simulink model "ADC_example1"  (Simulink 7.7)
settings: Solver=ode45  StartTime=0.0  StopTime=T  MaxStep=MaxStep  RelTol=RelTol
values from neighbouring files (symbols this model uses):
  J = 20    [initialization_exADC.m]
  rule = 1    [initialization_exADC.m]
  T = 10    [initialization_exADC.m]
  x0ADC = [0;0]    [initialization_exADC.m]
libraries: simulink x3
settings Model: Creator=pablonanez  LastModifiedBy=pablonanez

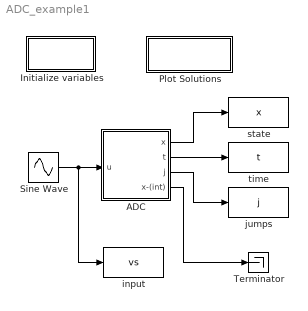
== system ADC_example1 ==
  ADC : Subsystem  LoadFcn=set_param(gcb,'LinkStatus','none')
      settings: CopyFcn=|
      | set_param(gcb,'LinkStatus','none'),
      | set_param(gcs, 'MaxStep', 'MaxStep', 'RelTol', 'RelTol','Stop time', 'T')
      mask Display:
      | image(imread('ADC.jpg'))
      | %plot([5 20 20 5 5],[5 5 20 20 5])
      | %text(8,13,'HyEq_mdl')
      | port_label('output', 1, 'x')
      | port_label('output', 2, 't')
      | port_label('output', 3, 'j')
      | port_label('output', 4, 'x-(int)')
      | port_label('input', 1, 'u')
  Initialize variables : Subsystem  Priority=-10
      settings: OpenFcn=initialization_exADC
      mask Display: disp('Double Click\n to Initialize')
  Plot Solutions : Subsystem
      settings: OpenFcn=postprocessing_exADC
      mask Display: disp('Double Click to\n Plot Solutions')
  Sine Wave : Sin  SampleTime=0
  Terminator : Terminator
  input : ToWorkspace  VariableName=vs  SampleTime=-1  SaveFormat=Array
  jumps : ToWorkspace  VariableName=j  SampleTime=-1  SaveFormat=Array
  state : ToWorkspace  VariableName=x  SampleTime=-1  SaveFormat=Array
  time : ToWorkspace  VariableName=t  SampleTime=-1  SaveFormat=Array
  wires:
  Sine Wave/1 -> ADC/1(u), input/1
  ADC/1(x) -> state/1
  ADC/2(t) -> time/1
  ADC/3(j) -> jumps/1
  ADC/4(x-(int)) -> Terminator/1

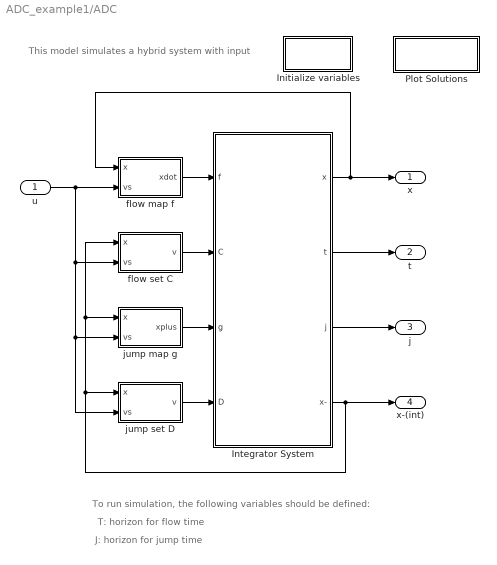
== system ADC_example1/ADC ==
  note: J: horizon for jump time
  note: T: horizon for flow time
  note: To run simulation, the following variables should be defined:
  note: This model simulates a hybrid system with input
  u : Inport
  Initialize variables : Subsystem  Priority=-10
      settings: OpenFcn=|
      | try
      |      clearvars -except inifile pathfile_in pathfile_pos posfile
      |      cd(pathfile_in);
      |      eval(inifile);
      | catch
      |      [inifile,pathfile_in] = getInitializationfile;
      |      cd(pathfile_in);
      |      inifile = strrep(inifile,'.m','');
      |      eval(inifile);
      | end
      mask Display: disp('Double Click\n to Initialize')
  Integrator System : Subsystem  Priority=2  mask(Hybrid Integrator){T=T, J=J, x0=x0ADC}
      mask prompts: T "Flow Horizon"; J "Jump Horizon"; x0 "Initial Condition"
      mask help:
      | This block integrates the state of the hybrid system defined by the flow map f (first input), the flow set C (second input), the jump map g (third input) and the jump set D (fourth input).
      | Starting from the initial condition x0 (last mask parameter), the system's state x evolves continuously within the set C, according to f(x,u), but is also subject to jumps within D, according to g(x,u).
      | The block also stops the simulation when the time t is greater than the flow horizon T (first mask parameter), or when the number of jumps j is greater than the jump horizon J (second mask parameter).
      | The outputs of the blocks are respectively x(t), t, j, x(t-).
      mask Help:
      | This block integrates the state of the hybrid system defined by the flow map f (first input), the flow set C (second input), the jump map g (third input) and the jump set D (fourth input).
      | <br>
      | Starting from the initial condition x0 (last mask parameter), the system's state x evolves continuously within the set C, according to f(x,u), but is also subject to jumps within D, according to g(x,u).
      | <br>
      | The block also stops the simulation when the time t is greater than the flow horizon T (first mask parameter), or when the number of jumps j is greater than the jump horizon J (second mask parameter).
      | <br>
      | The outputs of the blocks are respectively x(t), t, j, x(t-).
      | <br>
      | You can right click on the block and "Look under mask" to see what's inside the block.
      | Finally, refer to the manual (HybridSimulator_vXX.pdf) for more detailed information on how this hybrid simulator works.
  Plot Solutions : Subsystem
      settings: OpenFcn=|
      | try
      |      cd(pathfile_pos);
      |      eval(posfile);
      | catch
      |      [posfile,pathfile_pos] = getInitializationfile;
      |      cd(pathfile_pos);
      |      posfile = strrep(posfile,'.m','');
      |      eval(posfile);
      | end
      mask Display: disp('Double Click to\n Plot Solutions')
  flow map f : Stateflow chart  TreatAsAtomicUnit=on
  flow set C : Stateflow chart  TreatAsAtomicUnit=on
  jump map g : Stateflow chart  Priority=2  TreatAsAtomicUnit=on
  jump set D : Stateflow chart  TreatAsAtomicUnit=on
  x : Outport
  t : Outport  Port=2
  j : Outport  Port=3
  x-(int) : Outport  Port=4
  wires:
  jump map g/1(xplus) -> Integrator System/3(g)
  jump set D/1(v) -> Integrator System/4(D)
  u/1 -> jump set D/2(vs), jump map g/2(vs), flow set C/2(vs), flow map f/2(vs)
  Integrator System/3(j) -> j/1
  Integrator System/2(t) -> t/1
  flow set C/1(v) -> Integrator System/2(C)
  Integrator System/1(x) -> x/1, flow map f/1(x)
  Integrator System/4(x-) -> x-(int)/1, jump set D/1(x), flow set C/1(x), jump map g/1(x)
  flow map f/1(xdot) -> Integrator System/1(f)

== system ADC_example1/Initialize variables ==

== system ADC_example1/Plot Solutions ==

== system ADC_example1/ADC/Initialize variables ==

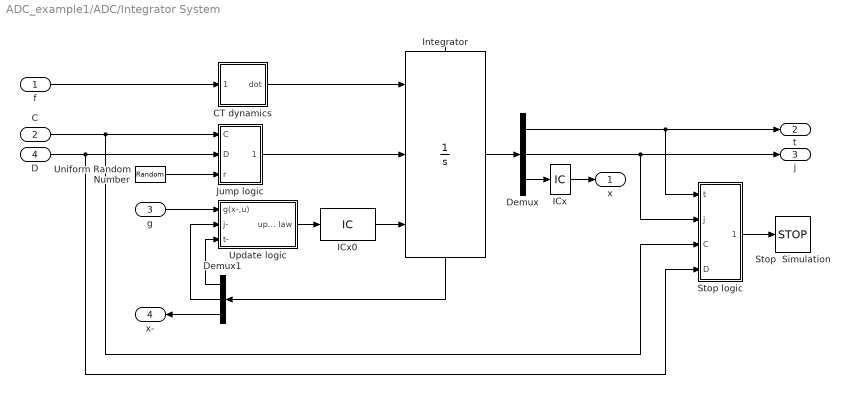
== system ADC_example1/ADC/Integrator System ==
  f : Inport
  C : Inport  Port=2
  g : Inport  Port=3
  D : Inport  Port=4
  CT dynamics : Subsystem
  Demux : Demux  Outputs=[1 1 -1]
  Demux1 : Demux  Outputs=[1 1 -1]
  ICx : InitialCondition  Value=x0
  ICx0 : InitialCondition  Value=[0; 0; x0(:)]
  Integrator : Integrator  ExternalReset=level hold  InitialConditionSource=external  ShowStatePort=on  ZeroCross=off
  Jump logic : Subsystem
  Stop  Simulation : Stop
  Stop logic : Subsystem
  Uniform Random Number : UniformRandomNumber  Minimum=0  Seed=abs(floor(100*rand))  SampleTime=0
  Update logic : Subsystem
  x : Outport
  t : Outport  Port=2
  j : Outport  Port=3
  x- : Outport  Port=4
  wires:
  ICx0/1 -> Integrator/3
  ICx/1 -> x/1
  Demux/3 -> ICx/1
  Integrator/State -> Demux1/1
  Demux/2 -> j/1, Stop logic/2(j)
  Demux/1 -> t/1, Stop logic/1(t)
  Update logic/1(update law) -> ICx0/1
  CT dynamics/1(dot) -> Integrator/1
  Stop logic/1(stop) -> Stop  Simulation/1
  Integrator/1 -> Demux/1
  C/1 -> Stop logic/3(C), Jump logic/1(C)
  D/1 -> Stop logic/4(D), Jump logic/2(D)
  f/1 -> CT dynamics/1(f(x,u))
  Demux1/3 -> x-/1
  Jump logic/1(jump) -> Integrator/2
  Uniform Random Number/1 -> Jump logic/3(r)
  g/1 -> Update logic/1(g(x-,u))
  Demux1/1 -> Update logic/3(t-)
  Demux1/2 -> Update logic/2(j-)

== system ADC_example1/ADC/Plot Solutions ==

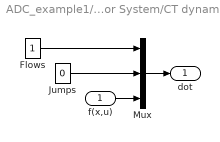
== system ADC_example1/ADC/Integrator System/CT dynamics ==
  f(x,u) : Inport
  Flows : Constant
  Jumps : Constant  Value=0
  Mux : Mux  Inputs=[1 1 -1]
  dot : Outport
  wires:
  Jumps/1 -> Mux/2
  Flows/1 -> Mux/1
  Mux/1 -> dot/1
  f(x,u)/1 -> Mux/3

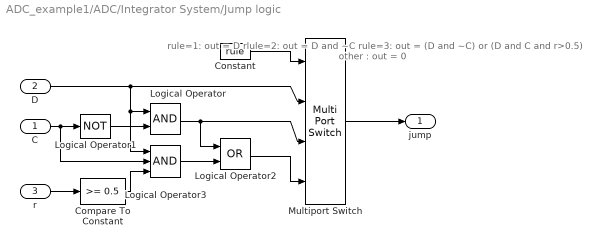
== system ADC_example1/ADC/Integrator System/Jump logic ==
  note: rule=1:  out = D
      | rlule=2: out = D and ~C
      | rule=3:  out = (D and ~C)  or (D and C and r>0.5)
      | other :  out = 0
  C : Inport
  D : Inport  Port=2
  r : Inport  Port=3
  Compare To Constant : simulink/Logic and Bit Operations/Compare To Constant  SystemSampleTime=-1  relop=>=  const=0.5  LogicOutDataTypeMode=uint8
  Constant : Constant  Value=rule
  Logical Operator : Logic  AllPortsSameDT=off  OutDataTypeStr=boolean
  Logical Operator1 : Logic  Operator=NOT  Inputs=1  AllPortsSameDT=off  OutDataTypeStr=boolean
  Logical Operator2 : Logic  Operator=OR  AllPortsSameDT=off  OutDataTypeStr=boolean
  Logical Operator3 : Logic  Inputs=3  AllPortsSameDT=off  OutDataTypeStr=boolean
  Multiport Switch : MultiPortSwitch  zeroidx=off
  jump : Outport
  wires:
  Constant/1 -> Multiport Switch/1
  D/1 -> Logical Operator3/1, Logical Operator/1, Multiport Switch/2
  r/1 -> Compare To Constant/1
  C/1 -> Logical Operator3/2, Logical Operator1/1
  Logical Operator1/1 -> Logical Operator/2
  Logical Operator/1 -> Multiport Switch/3, Logical Operator2/1
  Logical Operator2/1 -> Multiport Switch/4
  Multiport Switch/1 -> jump/1
  Compare To Constant/1 -> Logical Operator3/3
  Logical Operator3/1 -> Logical Operator2/2

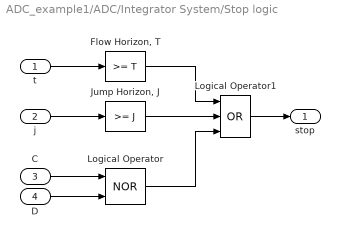
== system ADC_example1/ADC/Integrator System/Stop logic ==
  t : Inport
  j : Inport  Port=2
  C : Inport  Port=3
  D : Inport  Port=4
  "Flow Horizon, T" : simulink/Logic and Bit Operations/Compare To Constant  SystemSampleTime=-1  relop=>=  const=T  LogicOutDataTypeMode=uint8  ZeroCross=off
  "Jump Horizon, J" : simulink/Logic and Bit Operations/Compare To Constant  SystemSampleTime=-1  relop=>=  const=J  LogicOutDataTypeMode=uint8  ZeroCross=off
  Logical Operator : Logic  Operator=NOR  AllPortsSameDT=off  OutDataTypeStr=boolean
  Logical Operator1 : Logic  Operator=OR  Inputs=3  AllPortsSameDT=off  OutDataTypeStr=boolean
  stop : Outport
  wires:
  "Flow Horizon, T"/1 -> Logical Operator1/1
  "Jump Horizon, J"/1 -> Logical Operator1/2
  Logical Operator/1 -> Logical Operator1/3
  D/1 -> Logical Operator/2
  t/1 -> "Flow Horizon, T"/1
  j/1 -> "Jump Horizon, J"/1
  C/1 -> Logical Operator/1
  Logical Operator1/1 -> stop/1

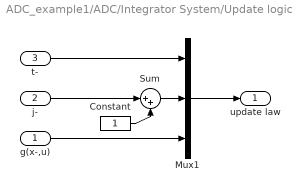
== system ADC_example1/ADC/Integrator System/Update logic ==
  g(x-,u) : Inport
  j- : Inport  Port=2
  t- : Inport  Port=3
  Constant : Constant
  Mux1 : Mux  Inputs=[1 1 -1]
  Sum : Sum  Inputs=|++
  update law : Outport
  wires:
  Sum/1 -> Mux1/2
  Mux1/1 -> update law/1
  j-/1 -> Sum/1
  g(x-,u)/1 -> Mux1/3
  t-/1 -> Mux1/1
  Constant/1 -> Sum/2

== matlab function ADC/flow map f ==
  data: x input double; xdot output double; vs input double
function xdot = f(x,vs)
%--------------------------------------------------------------------------
% Matlab M-file Project: HyEQ Toolbox @  Hybrid Systems Laboratory (HSL), 
% https://hybrid.soe.ucsc.edu/software
% http://hybridsimulator.wordpress.com/
%--------------------------------------------------------------------------
% Project: Simulation of a hybrid system Analog-to-Digital converter (ADC) 
% Description: Flow map
%--------------------------------------------------------------------------
%--------------------------------------------------------------------------
%   See also plotflows, plotHarc, plotHarcColor, plotHarcColor3D,
%   plotHybridArc, plotjumps.
%   Copyright @ Hybrid Systems Laboratory (HSL),
%   Revision: 0.0.0.3 Date: 05/20/2015 3:42:00

n = length(vs); % measured input size

msdot = zeros(n,1); % measured continuous dynamics
tau_sdot = 1; % Timer tau_s
xdot = [msdot;tau_sdot];

== matlab function ADC/flow set C ==
  data: x input double; v output double; vs input double; Ts parameter double
function v  = C(x, vs, Ts) 
%--------------------------------------------------------------------------
% Matlab M-file Project: HyEQ Toolbox @  Hybrid Systems Laboratory (HSL), 
% https://hybrid.soe.ucsc.edu/software
% http://hybridsimulator.wordpress.com/
%--------------------------------------------------------------------------
% Project: Simulation of a hybrid system Analog-to-Digital converter (ADC) 
% Description: Flow set
%--------------------------------------------------------------------------
%--------------------------------------------------------------------------
%   See also plotflows, plotHarc, plotHarcColor, plotHarcColor3D,
%   plotHybridArc, plotjumps.
%   Copyright @ Hybrid Systems Laboratory (HSL),
%   Revision: 0.0.0.3 Date: 05/20/2015 3:42:00
%
% Check on flow conditions
% E.g.,
% if (x(1) >= u(1))  % flow condition
%     v = 1;  % report flow
% else
%     v = 0;   % do not report flow
% end

n = length(vs); % measured input size

tau_s = x(end); % timer state

if tau_s>=0 && tau_s<= Ts
    v = 1; % report flow
elseif tau_s> Ts
    v = 0; % do not report flow
else
    v = 0;
end

== matlab function ADC/jump map g ==
  data: x input double; xplus output double; vs input double
function xplus = g(x, vs)
%--------------------------------------------------------------------------
% Matlab M-file Project: HyEQ Toolbox @  Hybrid Systems Laboratory (HSL), 
% https://hybrid.soe.ucsc.edu/software
% http://hybridsimulator.wordpress.com/
%--------------------------------------------------------------------------
% Project: Simulation of a hybrid system Analog-to-Digital converter (ADC) 
% Description: Jump map
%--------------------------------------------------------------------------
%--------------------------------------------------------------------------
%   See also plotflows, plotHarc, plotHarcColor, plotHarcColor3D,
%   plotHybridArc, plotjumps.
%   Copyright @ Hybrid Systems Laboratory (HSL),
%   Revision: 0.0.0.3 Date: 05/20/2015 3:42:00


n = length(vs); % measured input size

msplus = vs; % output = measured input
tau_splus = 0; % Timer tau_s
xplus = [msplus;tau_splus];

== matlab function ADC/jump set D ==
  data: x input double; v output double; vs input double; Ts parameter double
function v  = D(x, vs, Ts) 
%--------------------------------------------------------------------------
% Matlab M-file Project: HyEQ Toolbox @  Hybrid Systems Laboratory (HSL), 
% https://hybrid.soe.ucsc.edu/software
% http://hybridsimulator.wordpress.com/
%--------------------------------------------------------------------------
% Project: Simulation of a hybrid system Analog-to-Digital converter (ADC) 
% Description: Jump set
%--------------------------------------------------------------------------
%--------------------------------------------------------------------------
%   See also plotflows, plotHarc, plotHarcColor, plotHarcColor3D,
%   plotHybridArc, plotjumps.
%   Copyright @ Hybrid Systems Laboratory (HSL),
%   Revision: 0.0.0.3 Date: 05/20/2015 3:42:00
%
% Check on jump conditions
% % E.g.,
% if (x(1) <= u(1)) && (x(2) <= 0)  % jump condition
%     v = 1;  % report jump
% else
%     v = 0;   % do not report jump
% end

n = length(vs); % measured input size

tau_s = x(end); % timer state

if tau_s>=0 && tau_s<= Ts
    v = 0; % do not report jump
elseif tau_s> Ts
    v = 1; % report jump
else
    v = 0;
end
